simulink model "IMP2"  (R2017b)
settings: Solver=FixedStepAuto  StartTime=0.0  StopTime=sensorEndTime  FixedStep=0.0001  RelTol=1e-8
values from neighbouring files (symbols this model uses):
  K = 2    [IMP2_m.m]
libraries: cstblocks x3, simulink x1
settings Model: Creator=capn  LastModifiedBy=musin
settings CodeAppCC: StateflowObjectComments=on
settings SimscapeCC: SimscapeNormalizeSystem=off

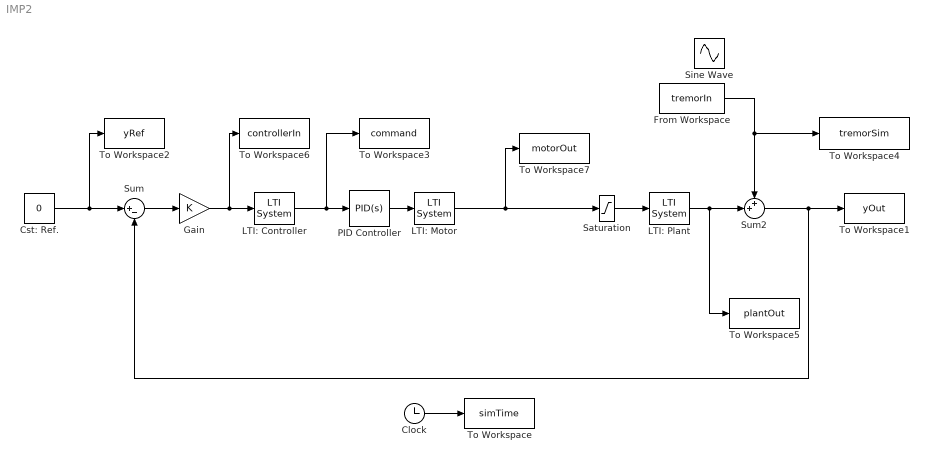
== system IMP2 ==
  Clock : Clock
  Cst: Ref. : Constant  Value=0
  From Workspace : FromWorkspace  VariableName=tremorIn  SampleTime=0
  Gain : Gain  Gain=K
  LTI: Controller : cstblocks/LTI System  sys=C  IC=[]
  LTI: Motor : cstblocks/LTI System  sys=M  IC=[]
  LTI: Plant : cstblocks/LTI System  sys=G  IC=[]
  PID Controller : simulink/Continuous/PID Controller  Controller=PID  TimeDomain=Continuous-time  SampleTime=-1  IntegratorMethod=Forward Euler  FilterMethod=Forward Euler  Form=Parallel  UseFilter=on  ControllerParametersSource=internal  P=10  I=0  D=1  N=100  InitialConditionSource=internal  InitialConditionForIntegrator=0  InitialConditionForFilter=0  ExternalReset=none  LimitOutput=off  UpperSaturationLimit=inf  LowerSaturationLimit=-inf  LinearizeAsGain=on  AntiWindupMode=none  Kb=1  TrackingMode=off  Kt=1  PParamMin=[]  PParamMax=[]  IParamMin=[]  IParamMax=[]  DParamMin=[]  DParamMax=[]  NParamMin=[]  NParamMax=[]  KbParamMin=[]  KbParamMax=[]  KtParamMin=[]  KtParamMax=[]  POutMin=[]  POutMax=[]  IOutMin=[]  IOutMax=[]  DOutMin=[]  DOutMax=[]  NOutMin=[]  NOutMax=[]  KbOutMin=[]  KbOutMax=[]  KtOutMin=[]  KtOutMax=[]  IntegratorOutMin=[]  IntegratorOutMax=[]  FilterOutMin=[]  FilterOutMax=[]  SumOutMin=[]  SumOutMax=[]  SumI1OutMin=[]  SumI1OutMax=[]  SumI2OutMin=[]  SumI2OutMax=[]  SumI3OutMin=[]  SumI3OutMax=[]  SumDOutMin=[]  SumDOutMax=[]  SaturationOutMin=[]  SaturationOutMax=[]  IntegratorContinuousStateAttributes=''  IntegratorStateMustResolveToSignalObject=off  IntegratorRTWStateStorageClass=Auto  FilterContinuousStateAttributes=''  FilterStateMustResolveToSignalObject=off  FilterRTWStateStorageClass=Auto  DifferentiatorICPrevScaledInput=0  DifferentiatorOutMin=[]  DifferentiatorOutMax=[]  InitialConditionSetting=State (most efficient)  FilterDiffOutCoefMin=[]  FilterDiffOutCoefMax=[]  SumDenOutMin=[]  SumDenOutMax=[]  SumNumOutMin=[]  SumNumOutMax=[]  ReciprocalOutMin=[]  ReciprocalOutMax=[]  DivideOutMin=[]  DivideOutMax=[]  TunerSelectOption=Transfer Function Based (PID Tuner App)
  Saturation : Saturate  UpperLimit=6.4  LowerLimit=-6.4
  Sine Wave : Sin  Amplitude=0.1  Frequency=5 * (2*pi)  SampleTime=0
  Sum : Sum  Inputs=|+-
  Sum2 : Sum  Inputs=++|
  To Workspace : ToWorkspace  VariableName=simTime  SampleTime=-1
  To Workspace1 : ToWorkspace  VariableName=yOut  SampleTime=-1
      settings: Save2DSignal=2-D array (concatenate along first dimension)
  To Workspace2 : ToWorkspace  VariableName=yRef  SampleTime=-1
      settings: Save2DSignal=2-D array (concatenate along first dimension)
  To Workspace3 : ToWorkspace  VariableName=command  SampleTime=-1
      settings: Save2DSignal=2-D array (concatenate along first dimension)
  To Workspace4 : ToWorkspace  VariableName=tremorSim  SampleTime=-1
      settings: Save2DSignal=2-D array (concatenate along first dimension)
  To Workspace5 : ToWorkspace  VariableName=plantOut  SampleTime=-1
      settings: Save2DSignal=2-D array (concatenate along first dimension)
  To Workspace6 : ToWorkspace  VariableName=controllerIn  SampleTime=-1
      settings: Save2DSignal=2-D array (concatenate along first dimension)
  To Workspace7 : ToWorkspace  VariableName=motorOut  SampleTime=-1
      settings: Save2DSignal=2-D array (concatenate along first dimension)
  wires:
  Sum/1 -> Gain/1
  Gain/1 -> LTI: Controller/1, To Workspace6/1
  Clock/1 -> To Workspace/1
  LTI: Plant/1 -> To Workspace5/1, Sum2/2
  Sum2/1 -> To Workspace1/1, Sum/2
  Cst: Ref./1 -> Sum/1, To Workspace2/1
  LTI: Controller/1 -> PID Controller/1, To Workspace3/1
  LTI: Motor/1 -> To Workspace7/1, Saturation/1
  PID Controller/1 -> LTI: Motor/1
  Saturation/1 -> LTI: Plant/1
  From Workspace/1 -> To Workspace4/1, Sum2/1
